simulink model "SubSystem_Container"  (R2023b)
settings: Solver=VariableStepAuto  StartTime=0.0  StopTime=10.0  RelTol=1e-3
settings Model: Creator=pkesarwa  LastModifiedBy=pkesarwa

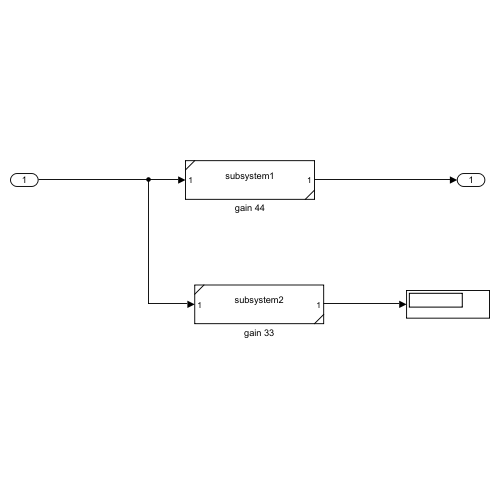
[thumbnail: Simulink's stored preview of the top-level diagram]
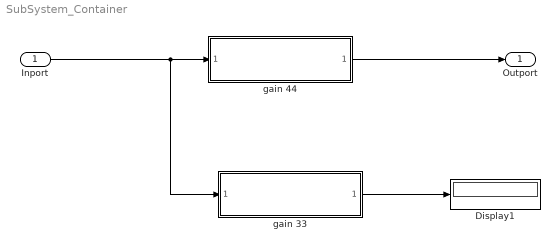
== system SubSystem_Container ==
  Inport : Inport
  Display1 : Display
  gain 33 : Subsystem  ReferencedSubsystem=subsystem2
  gain 44 : Subsystem  ReferencedSubsystem=subsystem1
  Outport : Outport
  wires:
  Inport/1 -> gain 33/1, gain 44/1
  gain 44/1 -> Outport/1
  gain 33/1 -> Display1/1
